simulink model "simulink_221036"  (R2022b)
settings: Solver=VariableStepAuto  StartTime=0.0  StopTime=10.0  RelTol=1e-3
settings Model: Creator=Admin200  LastModifiedBy=Admin200

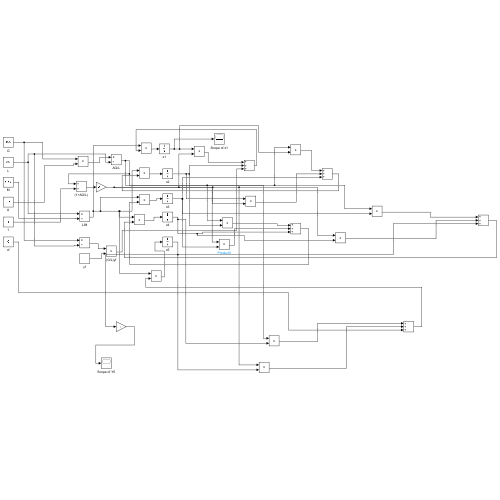
[thumbnail: Simulink's stored preview of the top-level diagram]
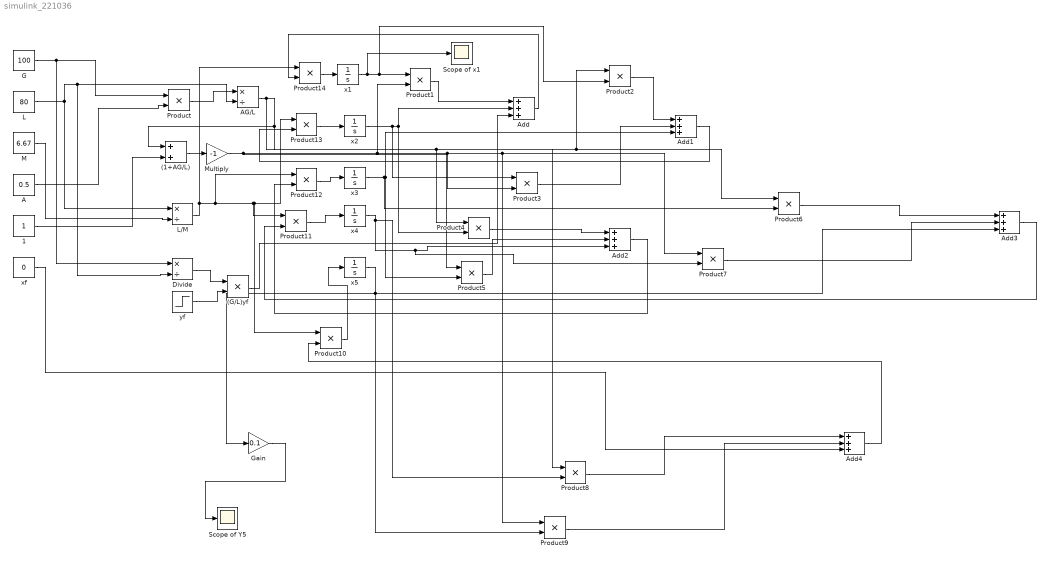
== system simulink_221036 ==
  (1+AG/L) : Sum
  (G/L)yf : Product
  1 : Constant
  A : Constant  Value=0.5
  AG/L : Product  Inputs=*/
  Add{,1..4} (5 alike) : Sum  Inputs=+++
  Divide : Product  Inputs=*/
  G : Constant  Value=100
  Gain : Gain  Gain=0.1
  L : Constant  Value=80
  L/M : Product  Inputs=*/
  M : Constant  Value=6.67
  Multiply : Gain  Gain=-1
  Product{,1..14} (15 alike) : Product
  Scope of Y5 : Scope
  Scope of x1 : Scope
  x1 : Integrator  InitialCondition=0.1202
  x2 : Integrator  InitialCondition=0.0704
  x3 : Integrator  InitialCondition=0.0392
  x4 : Integrator  InitialCondition=0.0198
  x5 : Integrator  InitialCondition=0.0076
  xf : Constant  Value=0
  yf : Step  Time=0  Before=0.1  After=0.15  SampleTime=0
  wires:
  G/1 -> Divide/1, Product/1
  A/1 -> Product/2
  Product/1 -> AG/L/1
  L/1 -> L/M/1, Divide/2, AG/L/2
  1/1 -> (1+AG/L)/2
  AG/L/1 -> Product8/1, Product2/1, Product6/1, Product4/1, (1+AG/L)/1
  M/1 -> L/M/2
  yf/1 -> (G/L)yf/2
  Divide/1 -> (G/L)yf/1
  (1+AG/L)/1 -> Multiply/1
  Multiply/1 -> Product9/1, Product7/1, Product3/2, Product1/2, Product5/1
  x1/1 -> Scope of x1/1, Product2/2, Product1/1
  Product1/1 -> Add/1
  x2/1 -> Product3/1, Product4/2, Add/2
  (G/L)yf/1 -> Add/3
  Product2/1 -> Add1/1
  Product3/1 -> Add1/2
  x3/1 -> Product6/2, Product5/2, Add1/3
  Product4/1 -> Add2/1
  Product5/1 -> Add2/2
  x4/1 -> Product8/2, Product7/2, Add2/3
  Product6/1 -> Add3/1
  Product7/1 -> Add3/2
  x5/1 -> Gain/1, Product9/2, Add3/3
  Product8/1 -> Add4/1
  Product9/1 -> Add4/2
  xf/1 -> Add4/3
  L/M/1 -> Product12/1, Product10/1, Product13/1, Product11/1, Product14/1
  Add/1 -> Product14/2
  Product14/1 -> x1/1
  Add1/1 -> Product13/2
  Product13/1 -> x2/1
  Add2/1 -> Product12/2
  Product12/1 -> x3/1
  Add3/1 -> Product11/2
  Product11/1 -> x4/1
  Add4/1 -> Product10/2
  Product10/1 -> x5/1
  Gain/1 -> Scope of Y5/1
